simulink model "tutorial30_suspension"  (R2025a)
settings: Solver=VariableStepAuto  StartTime=0.0  StopTime=10.0  RelTol=1e-3
settings Model: Creator=xing2  LastModifiedBy=xing2

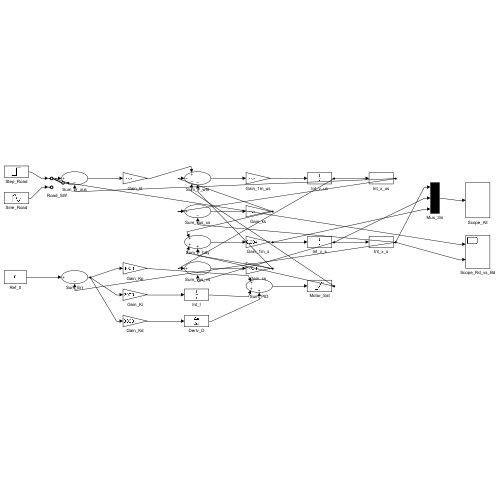
[thumbnail: Simulink's stored preview of the top-level diagram]
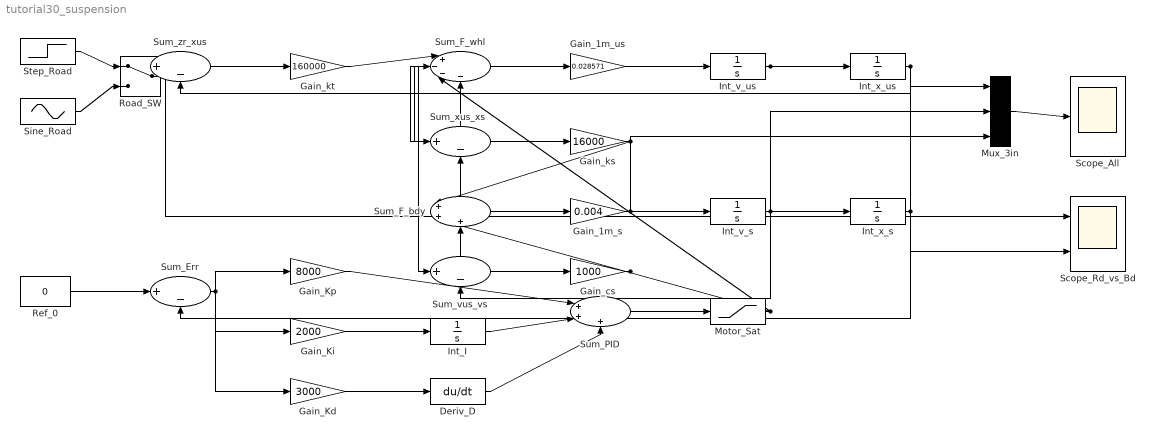
== system tutorial30_suspension ==
  Deriv_D : Derivative
  Gain_1m_s : Gain  Gain=0.004
  Gain_1m_us : Gain  Gain=0.028571
  Gain_Kd : Gain  Gain=3000
  Gain_Ki : Gain  Gain=2000
  Gain_Kp : Gain  Gain=8000
  Gain_cs : Gain  Gain=1000
  Gain_ks : Gain  Gain=16000
  Gain_kt : Gain  Gain=160000
  Int_I : Integrator
  Int_v_s : Integrator
  Int_v_us : Integrator
  Int_x_s : Integrator
  Int_x_us : Integrator
  Motor_Sat : Saturate  UpperLimit=2000  LowerLimit=-2000
  Mux_3in : Mux  Inputs=3
  Ref_0 : Constant  Value=0
  Road_SW : ManualSwitch
  Scope_All : Scope
  Scope_Rd_vs_Bd : Scope  NumInputPorts=2
  Sine_Road : Sin  Amplitude=0.03  Frequency=6.28  SampleTime=0
  Step_Road : Step  Time=0.5  After=0.05  SampleTime=0
  Sum_Err : Sum  Inputs=|+-
  Sum_F_bdy : Sum  Inputs=|+++
  Sum_F_whl : Sum  Inputs=|+---
  Sum_PID : Sum  Inputs=|+++
  Sum_vus_vs : Sum  Inputs=|+-
  Sum_xus_xs : Sum  Inputs=|+-
  Sum_zr_xus : Sum  Inputs=|+-
  wires:
  Step_Road/1 -> Road_SW/1
  Sine_Road/1 -> Road_SW/2
  Road_SW/1 -> Sum_zr_xus/1, Scope_Rd_vs_Bd/1
  Sum_zr_xus/1 -> Gain_kt/1
  Gain_kt/1 -> Sum_F_whl/1
  Sum_F_whl/1 -> Gain_1m_us/1
  Gain_1m_us/1 -> Int_v_us/1
  Int_v_us/1 -> Int_x_us/1, Sum_vus_vs/1
  Int_x_us/1 -> Sum_zr_xus/2, Sum_xus_xs/1
  Sum_xus_xs/1 -> Gain_ks/1
  Gain_ks/1 -> Sum_F_whl/2, Sum_F_bdy/1
  Sum_F_bdy/1 -> Gain_1m_s/1
  Gain_1m_s/1 -> Int_v_s/1, Mux_3in/3
  Int_v_s/1 -> Int_x_s/1, Sum_vus_vs/2, Mux_3in/2
  Int_x_s/1 -> Sum_xus_xs/2, Sum_Err/2, Mux_3in/1, Scope_Rd_vs_Bd/2
  Sum_vus_vs/1 -> Gain_cs/1
  Gain_cs/1 -> Sum_F_whl/4, Sum_F_bdy/3
  Ref_0/1 -> Sum_Err/1
  Sum_Err/1 -> Gain_Kp/1, Gain_Ki/1, Gain_Kd/1
  Gain_Ki/1 -> Int_I/1
  Gain_Kd/1 -> Deriv_D/1
  Gain_Kp/1 -> Sum_PID/1
  Int_I/1 -> Sum_PID/2
  Deriv_D/1 -> Sum_PID/3
  Sum_PID/1 -> Motor_Sat/1
  Motor_Sat/1 -> Sum_F_bdy/2, Sum_F_whl/3
  Mux_3in/1 -> Scope_All/1
